simulink model "El_control_del_charlo"  (R2018a)
settings: Solver=VariableStepAuto  StartTime=0.0  StopTime=40  RelTol=1e-3
PreLoadFcn:
  | EJ2_init;
InitFcn:
  | EJ2_init;
StartFcn:
  | hold on;
  | patch([2 0 0 2],[0 2 2 0], [-2 -2 1 1],'g' );
undefined symbols (not defined in the file or in its folder): cfg
libraries: simulink x1, roblocks x1
CloseFcn:
  | hold off;
settings Model: Creator=Guido L  LastModifiedBy=Guido L

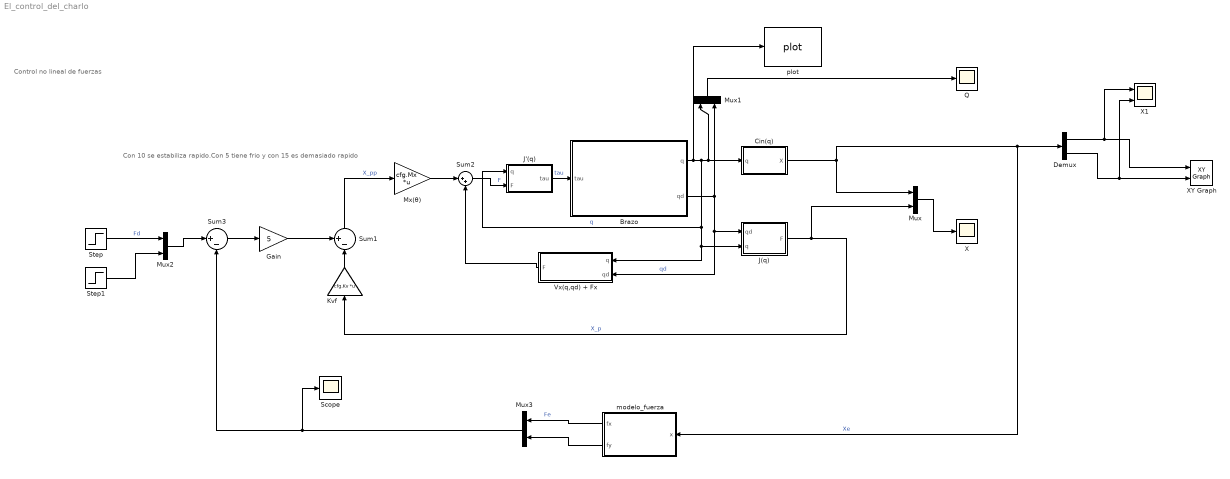
== system El_control_del_charlo ==
  note: Con 10 se estabiliza rapido.Con 5 tiene frio y con 15 es demasiado rapido
  note: Control no lineal de fuerzas
  Brazo : Subsystem
      mask Display: image('juan.jpg');
  Cin(q) : Subsystem
  Demux : Demux  Outputs=2
  Gain : Gain  Gain=5
  J'(q) : Subsystem
  J(q) : Subsystem
  Kvf : Gain  Gain=cfg.Kv  Multiplication=Matrix(K*u) (u vector)
  Mux{,1..3} (4 alike) : Mux  Inputs=2
  "Mx(θ) " : Gain  Gain=cfg.Mx  Multiplication=Matrix(K*u) (u vector)
  Q : Scope
  Scope : Scope
  Step : Step  After=10  SampleTime=0
  Step1 : Step  After=10  SampleTime=0
  Sum1 : Sum  Inputs=+-|
  Sum2 : Sum  Inputs=|++
  Sum3 : Sum  Inputs=|+-
  Vx(q,qd) + Fx : Subsystem
  X : Scope
  X1 : Scope  NumInputPorts=2
  XY Graph : simulink/Sinks/XY Graph  xmin=-2  xmax=2  ymin=-2  ymax=2  st=-1
  modelo_fuerza : MATLAB Function  TreatAsAtomicUnit=on
  plot : roblocks/Arm/plot  robot=Juan  fps=10  holdplot=on
  wires:
  Demux/2 -> X1/2, XY Graph/2
  Demux/1 -> X1/1, XY Graph/1
  Brazo/1(q) -> plot/1, Mux1/1, Cin(q)/1(q), J(q)/2(q), Vx(q,qd) + Fx/1(q), J'(q)/2(q)  "q"
  Mux1/1 -> Q/1
  Vx(q,qd) + Fx/1(F) -> Sum2/2
  Cin(q)/1(X) -> Mux/1, modelo_fuerza/1(x), Demux/1  "Xe"
  Mux/1 -> X/1
  J(q)/1(F) -> Kvf/1, Mux/2  "X_p"
  Sum1/1 -> "Mx(θ) "/1  "X_pp"
  "Mx(θ) "/1 -> Sum2/1
  Sum2/1 -> J'(q)/1(F)  "F"
  Brazo/2(qd) -> Vx(q,qd) + Fx/2(qd), J(q)/1(qd), Mux1/2  "qd"
  J'(q)/1(tau) -> Brazo/1(tau)  "tau"
  Kvf/1 -> Sum1/2
  Step/1 -> Mux2/1  "Fd"
  Sum3/1 -> Gain/1
  Gain/1 -> Sum1/1
  Step1/1 -> Mux2/2
  Mux2/1 -> Sum3/1
  modelo_fuerza/2(fy) -> Mux3/2
  modelo_fuerza/1(fx) -> Mux3/1  "Fe"
  Mux3/1 -> Scope/1, Sum3/2

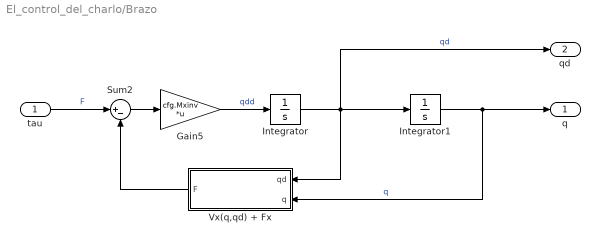
== system El_control_del_charlo/Brazo ==
  tau : Inport
  Gain5 : Gain  Gain=cfg.Mxinv  Multiplication=Matrix(K*u) (u vector)
  Integrator : Integrator  InitialCondition=[0 0]
  Integrator1 : Integrator  InitialCondition=[pi/2 0 ]
  Sum2 : Sum  Inputs=|+-
  Vx(q,qd) + Fx : Subsystem
  q : Outport  VectorParamsAs1DForOutWhenUnconnected=on
  qd : Outport  Port=2  VectorParamsAs1DForOutWhenUnconnected=on
  wires:
  Gain5/1 -> Integrator/1  "qdd"
  Integrator/1 -> Vx(q,qd) + Fx/1(qd), Integrator1/1, qd/1  "qd"
  tau/1 -> Sum2/1  "F"
  Sum2/1 -> Gain5/1
  Integrator1/1 -> Vx(q,qd) + Fx/2(q), q/1  "q"
  Vx(q,qd) + Fx/1(F) -> Sum2/2

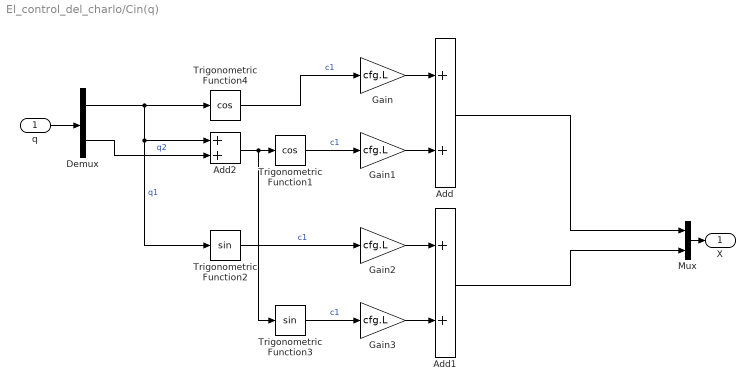
== system El_control_del_charlo/Cin(q) ==
  q : Inport
  Add : Sum
  Add1 : Sum
  Add2 : Sum
  Demux : Demux  Outputs=2
  Gain{,1..3} (4 alike) : Gain  Gain=cfg.L
  Mux : Mux  Inputs=2
  Trigonometric Function1 : Trigonometry  Operator=cos
  Trigonometric Function2 : Trigonometry
  Trigonometric Function3 : Trigonometry
  Trigonometric Function4 : Trigonometry  Operator=cos
  X : Outport  VectorParamsAs1DForOutWhenUnconnected=on
  wires:
  Demux/1 -> Trigonometric Function2/1, Add2/1, Trigonometric Function4/1  "q1"
  q/1 -> Demux/1
  Mux/1 -> X/1
  Trigonometric Function4/1 -> Gain/1  "c1"
  Gain/1 -> Add/1
  Demux/2 -> Add2/2  "q2"
  Add2/1 -> Trigonometric Function3/1, Trigonometric Function1/1
  Trigonometric Function1/1 -> Gain1/1  "c1"
  Add/1 -> Mux/1
  Gain1/1 -> Add/2
  Trigonometric Function2/1 -> Gain2/1  "c1"
  Gain2/1 -> Add1/1
  Gain3/1 -> Add1/2
  Trigonometric Function3/1 -> Gain3/1  "c1"
  Add1/1 -> Mux/2

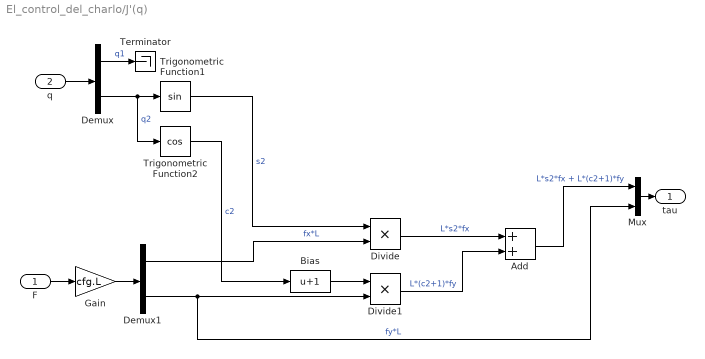
== system El_control_del_charlo/J'(q) ==
  F : Inport
  q : Inport  Port=2
  Add : Sum
  Bias : Bias  Bias=1
  Demux : Demux  Outputs=2
  Demux1 : Demux  Outputs=2
  Divide : Product  Inputs=**
  Divide1 : Product  Inputs=**
  Gain : Gain  Gain=cfg.L
  Mux : Mux  Inputs=2
  Terminator : Terminator
  Trigonometric Function1 : Trigonometry
  Trigonometric Function2 : Trigonometry  Operator=cos
  tau : Outport  VectorParamsAs1DForOutWhenUnconnected=on
  wires:
  Demux/2 -> Trigonometric Function2/1, Trigonometric Function1/1  "q2"
  Demux/1 -> Terminator/1  "q1"
  q/1 -> Demux/1
  Trigonometric Function1/1 -> Divide/1  "s2"
  Trigonometric Function2/1 -> Bias/1  "c2"
  Demux1/1 -> Divide/2  "fx*L"
  Demux1/2 -> Mux/2, Divide1/2  "fy*L"
  Mux/1 -> tau/1
  F/1 -> Gain/1
  Gain/1 -> Demux1/1
  Divide/1 -> Add/1  "L*s2*fx"
  Bias/1 -> Divide1/1
  Divide1/1 -> Add/2  "L*(c2+1)*fy"
  Add/1 -> Mux/1  "L*s2*fx + L*(c2+1)*fy"

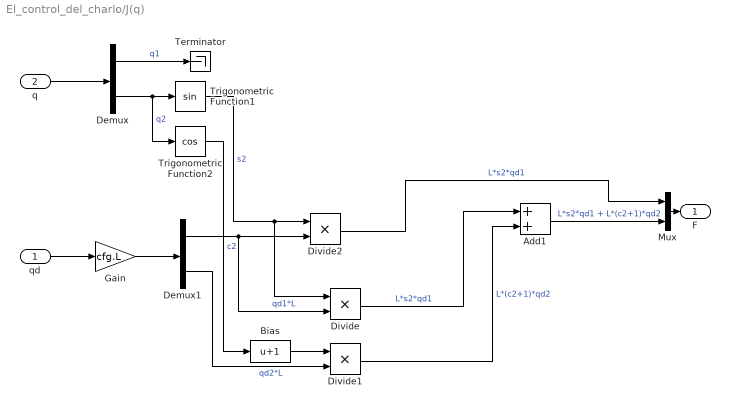
== system El_control_del_charlo/J(q) ==
  qd : Inport
  q : Inport  Port=2
  Add1 : Sum
  Bias : Bias  Bias=1
  Demux : Demux  Outputs=2
  Demux1 : Demux  Outputs=2
  Divide : Product  Inputs=**
  Divide1 : Product  Inputs=**
  Divide2 : Product  Inputs=**
  Gain : Gain  Gain=cfg.L
  Mux : Mux  Inputs=2
  Terminator : Terminator
  Trigonometric Function1 : Trigonometry
  Trigonometric Function2 : Trigonometry  Operator=cos
  F : Outport  VectorParamsAs1DForOutWhenUnconnected=on
  wires:
  Divide1/1 -> Add1/2  "L*(c2+1)*qd2"
  Divide/1 -> Add1/1  "L*s2*qd1"
  q/1 -> Demux/1
  Bias/1 -> Divide1/1
  Demux/2 -> Trigonometric Function2/1, Trigonometric Function1/1  "q2"
  Gain/1 -> Demux1/1
  Mux/1 -> F/1
  Demux/1 -> Terminator/1  "q1"
  qd/1 -> Gain/1
  Add1/1 -> Mux/2  "L*s2*qd1 + L*(c2+1)*qd2"
  Demux1/1 -> Divide/2, Divide2/2  "qd1*L"
  Trigonometric Function1/1 -> Divide/1, Divide2/1  "s2"
  Divide2/1 -> Mux/1  "L*s2*qd1"
  Demux1/2 -> Divide1/2  "qd2*L"
  Trigonometric Function2/1 -> Bias/1  "c2"

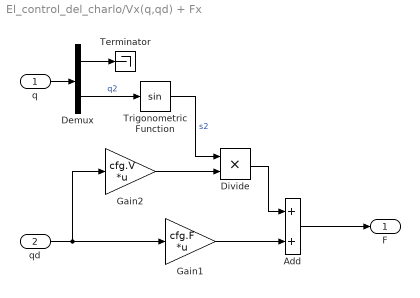
== system El_control_del_charlo/Vx(q,qd) + Fx ==
  q : Inport
  qd : Inport  Port=2
  Add : Sum
  Demux : Demux  Outputs=2
  Divide : Product  Inputs=**
  Gain1 : Gain  Gain=cfg.F  Multiplication=Matrix(K*u) (u vector)
  Gain2 : Gain  Gain=cfg.V  Multiplication=Matrix(K*u) (u vector)
  Terminator : Terminator
  Trigonometric Function : Trigonometry
  F : Outport  VectorParamsAs1DForOutWhenUnconnected=on
  wires:
  qd/1 -> Gain1/1, Gain2/1
  Gain1/1 -> Add/2
  Add/1 -> F/1
  Gain2/1 -> Divide/2
  q/1 -> Demux/1
  Demux/1 -> Terminator/1
  Demux/2 -> Trigonometric Function/1  "q2"
  Divide/1 -> Add/1
  Trigonometric Function/1 -> Divide/1  "s2"

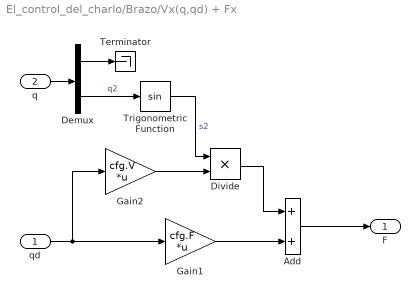
== system El_control_del_charlo/Brazo/Vx(q,qd) + Fx ==
  qd : Inport
  q : Inport  Port=2
  Add : Sum
  Demux : Demux  Outputs=2
  Divide : Product  Inputs=**
  Gain1 : Gain  Gain=cfg.F  Multiplication=Matrix(K*u) (u vector)
  Gain2 : Gain  Gain=cfg.V  Multiplication=Matrix(K*u) (u vector)
  Terminator : Terminator
  Trigonometric Function : Trigonometry
  F : Outport  VectorParamsAs1DForOutWhenUnconnected=on
  wires:
  qd/1 -> Gain1/1, Gain2/1
  Gain1/1 -> Add/2
  Add/1 -> F/1
  Gain2/1 -> Divide/2
  q/1 -> Demux/1
  Demux/1 -> Terminator/1
  Demux/2 -> Trigonometric Function/1  "q2"
  Divide/1 -> Add/1
  Trigonometric Function/1 -> Divide/1  "s2"

== matlab function El_control_del_charlo/modelo_fuerza ==
  data: x input; fx output; fy output
function [fx, fy] = modelo_fuerza(x)
    %La idea es que esto devuelva la reaccion que tiene la pared sobre el
    %end efector cuando este le aplica presión por lo tanto hasta que no
    %choque con la misma no devolvera ningun valor de fuerza
wall.m=-1;%pendiente de la funcion que describe la pared
wall.b=2;%ordenada a origen de la misma
wall.ke=1000;%coeficiente de rigidez del cuerpo rigido, del modelo f=ke*x\

     x_ee=x(1);
     y_ee=x(2);
     y_pared=wall.m*x_ee+wall.b;
     x_pared= (y_ee-wall.b)/wall.m;
     if((y_ee < y_pared )&&(x_ee < x_pared))%Si no me choque con la pared no hago fuerza
         f=0;
     else
     dist = abs(wall.m*x_ee+2-y_ee)/sqrt(wall.m^2+1); %esto describe la distancia entre la posicion
%     del end efector y la pared por el camino mas corto (Linea ortogonal a la superficie de la pared)
     f=wall.ke*dist;%calculo de la fuerza segun el modelo de rigidez
     end
     fx= f/sqrt(2);
     fy = fx;         

end
